simulink model "Closed_loop_Interferometer_v6_multiple_setpoint"  (R2019b)
settings: Solver=ode3  StartTime=0.0  StopTime=0.1  FixedStep=0.000001  RelTol=1e-3  EnableMultiTasking=on
InitFcn:
  | %clear all
  | %close all
  | clc
  | 
  | vmax = 8.87;
  | vmin = 1.25;
  | 
  | A = (vmax+vmin)/2;
  | V = (vmax-vmin)/(vmax+vmin);
  | 
  | timer= 0.1;
StopFcn:
  | set(groot,'defaultAxesTickLabelInterpreter','latex')
  | set(groot,'defaultLegendInterpreter','latex')
  | xc = 0.3;
  | 
  | %%%%
  | figure('Units','centimeter','Position',[0 0 20 30])
  | 
  | 
  | subplot(6,1,1)
  | plot(cleanSignal,'Color',[xc,xc,xc])
  | xlim([0 inf])
  | %ylim([-1 1])
  | xlabel('Time [s]','Interpreter','latex', 'FontSize', 10)
  | ylabel({'Input signal' ;'[rad]'},'Interpreter','latex', 'FontSize', 10)
  | title('')
  | grid
  | 
  | subplot(6,1,2)
  | plot(input,'Color',[xc,xc,xc])
  | %ylim([0.8*min(input.data) 1.2*max(input.data)])
  | xlim([0 inf])
  | xlabel('Time [s]','Interpreter','latex', 'FontSize', 10)
  | ylabel({'Input signal w/';'disturbances [rad]'},'Interpreter','latex', 'FontSize', 10)
  | title('')
  | grid
  | 
  | 
  | subplot(6,1,3)
  | plot(signFunc,'Color',[xc,xc,xc],'LineWidth',0.1)
  | ylim([-1.2 1.2])
  | xlim([0 inf])
  | xlabel('Time [s]','Interpreter','latex', 'FontSize', 10)
  | ylabel({'Sign function';'output [V]'},'Interpreter','latex', 'FontSize', 10)
  | title('')
  | grid
  | 
  | 
  | subplot(6,1,4)
  | plot(controlSignal,'Color',[xc,xc,xc])
  | %ylim([-5 0.2])
  | xlim([0 inf])
  | xlabel('Time [s]','Interpreter','latex', 'FontSize', 10)
  | ylabel({'Feedback control';'signal [rad]' },'Interpreter','latex', 'FontSize', 10)
  | title('')
  | grid minor
  | 
  | subplot(6,1,5)
  | plot(output2,'Color',[xc,xc,xc])
  | hold on
  | yline(A+A*V);
  | yline(A-A*V);
  | ylim([0 10])
  | xlim([0 inf])
  | xlabel('Time [s]','Interpreter','latex', 'FontSize', 10)
  | ylabel('Output [V]' ,'Interpreter','latex', 'FontSize', 10)
  | title('')
  | grid minor
  | 
  | fig = figure('Units','centimeter','Position',[0 1 6.5*1.4 6.5],...
  |         'PaperPositionMode','auto')
  | hold on
  | ylim([0 10])
  | xlim([90 100])
  | ylabel('Output [V]', 'interpreter','latex')
  | xlabel('Time [s]', 'interpreter','latex')
  | yline(A+A*V,'color',[.7 .7 .7]);
  | yline(A-A*V,'color',[.7 .7 .7]);
  | title('')
  | plot(output2.Time*1000,output2.Data)
  | ticks = get(gca,'Xtick');
  | newticks = ticks-ticks(1)
  | set(gca, 'Xticklabel', strsplit(num2str(newticks)))
  | box on
  | 
  | sp2v = output2;
  | 
  | 
  | %figure
  | %plot(lowpass,'Color',[xc,xc,xc])
  | 
  | %cd 'D:\Users\Stinky\Google Drive\ITA\Codes\MATLAB'
  | 
  | %print('test','-dpdf'); %-dpng , -depsc, -tiff, -dpdf
undefined symbols (not defined in the file or in its folder): sgn
libraries: simulink x1, dsparch4 x1
settings Model: Creator=Roberta Martin  LastModifiedBy=Stinky
settings DataIOCC: LimitDataPoints=on  SaveFormat=Array  ReturnWorkspaceOutputs=off
settings OptimizationCC: LifeSpan=inf
settings DebuggingCC: UnderspecifiedInitializationDetection=Classic  MergeDetectMultiDrivingBlocksExec=none  SolverPrmCheckMsg=warning  AllowSymbolicDim=off  SFUnexpectedBacktrackingDiag=warning  SFNoUnconditionalDefaultTransitionDiag=warning  SFExecutionAtInitializationDiag=none  ArithmeticOperatorsInVariantConditions=warning
settings HardwareCC: ProdBitPerPointer=32  ProdBitPerSizeT=32  ProdBitPerPtrDiffT=32  ProdLargestAtomicFloat=None  ProdIntDivRoundTo=Undefined  ProdEndianess=Unspecified  ProdWordSize=32  ProdHWDeviceType=32-bit Generic
settings ModelReferenceCC: PropagateSignalLabelsOutOfModel=off
settings SFSimCC: SimUseLocalCustomCode=off  CustomCodeUndefinedFunction=UseInterfaceOnly
settings RTWCC: RTWUseLocalCustomCode=off
settings CodeAppCC: StateflowObjectComments=on
settings GRTTargetCC: TargetLangStandard=C89/C90 (ANSI)  GeneratePreprocessorConditionals=Disable all
settings ConfigComp: CovMetricSettings=dw  CovHtmlReporting=on  CovSaveCumulativeToWorkspaceVar=on  CovSaveSingleToWorkspaceVar=on  CovExternalEMLEnable=off
settings SimscapeCC: SimscapeNormalizeSystem=off

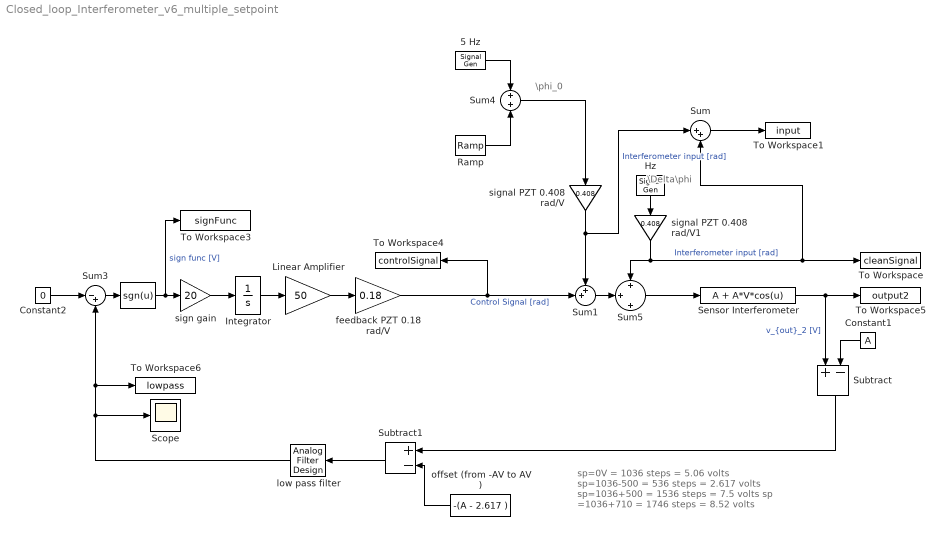
== system Closed_loop_Interferometer_v6_multiple_setpoint ==
  note: sp=0V = 1036 steps = 5.06 volts
      | sp=1036-500 = 536 steps = 2.617 volts
      | sp=1036+500 = 1536 steps =  7.5 volts
      | sp =1036+710 = 1746 steps = 8.52 volts
  note: \phi_0
  note: \Delta\phi
  " " : Fcn  Expr=sgn(u)
  " 5 Hz" : SignalGenerator  Amplitude=2  Frequency=5
  Constant1 : Constant  Value=A
  Constant2 : Constant  Value=0
  "Hz " : SignalGenerator  Amplitude=0.75  Frequency=500
  Integrator : Integrator  UpperSaturationLimit=15  LowerSaturationLimit=-15
  Linear Amplifier : Gain  Gain=50
  Ramp : simulink/Sources/Ramp  slope=10  start=0  InitialOutput=0
  Scope : Scope
  Sensor Interferometer : Fcn  Expr=A + A*V*cos(u)
  Subtract : Sum  Inputs=+-
  Subtract1 : Sum  Inputs=+-
  Sum : Sum  Inputs=|++
  Sum1 : Sum  Inputs=++|
  Sum3 : Sum  Inputs=|-+
  Sum4 : Sum  Inputs=+|+
  Sum5 : Sum  Inputs=+|+|+
  To Workspace : ToWorkspace  VariableName=cleanSignal  SaveFormat=Timeseries  SampleTime=-1
  To Workspace1 : ToWorkspace  VariableName=input  SaveFormat=Timeseries  SampleTime=-1
  To Workspace3 : ToWorkspace  VariableName=signFunc  SaveFormat=Timeseries  SampleTime=-1
  To Workspace4 : ToWorkspace  VariableName=controlSignal  SaveFormat=Timeseries  SampleTime=-1
  To Workspace5 : ToWorkspace  VariableName=output2  SaveFormat=Timeseries  SampleTime=-1
  To Workspace6 : ToWorkspace  VariableName=lowpass  SaveFormat=Timeseries  SampleTime=-1
  feedback PZT 0.18 rad/V : Gain  Gain=0.18
  low pass filter : dsparch4/Analog Filter Design  method=Butterworth  filttype=Lowpass  N=1  Wlo=1000*2*pi  Whi=80  Rp=2  Rs=40
  offset (from -AV to AV ) : Constant  Value=-(A - 2.617 )  VectorParams1D=off
  sign gain : Gain  Gain=20
  signal PZT 0.408 rad/V : Gain  Gain=0.408
  signal PZT 0.408 rad/V1 : Gain  Gain=0.408
  wires:
  Sum1/1 -> Sum5/2
  Linear Amplifier/1 -> feedback PZT 0.18 rad/V/1
  signal PZT 0.408 rad/V/1 -> Sum/1, Sum1/1  "Interferometer input [rad]"
  Sum3/1 -> " "/1
  Constant2/1 -> Sum3/1
  sign gain/1 -> Integrator/1
  " 5 Hz"/1 -> Sum4/1
  Ramp/1 -> Sum4/2
  " "/1 -> To Workspace3/1, sign gain/1  "sign func [V]"
  Integrator/1 -> Linear Amplifier/1
  Sensor Interferometer/1 -> Subtract/1, To Workspace5/1  "v_{out}_2 [V]"
  low pass filter/1 -> To Workspace6/1, Sum3/2, Scope/1
  Sum4/1 -> signal PZT 0.408 rad/V/1
  "Hz "/1 -> signal PZT 0.408 rad/V1/1
  signal PZT 0.408 rad/V1/1 -> To Workspace/1, Sum/2, Sum5/1  "Interferometer input [rad]"
  feedback PZT 0.18 rad/V/1 -> To Workspace4/1, Sum1/2  "Control Signal [rad]"
  Constant1/1 -> Subtract/2
  Subtract/1 -> Subtract1/1
  offset (from -AV to AV )/1 -> Subtract1/2
  Subtract1/1 -> low pass filter/1
  Sum5/1 -> Sensor Interferometer/1
  Sum/1 -> To Workspace1/1
